simulink model "wychladzanie_obiektu"  (R2020b)
settings: Solver=VariableStepAuto  StartTime=0.0  StopTime=60  RelTol=1e-3
settings Model: Creator=matis  LastModifiedBy=matis

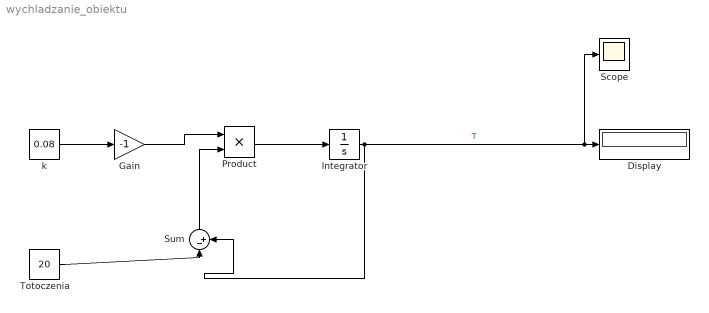
== system wychladzanie_obiektu ==
  Display : Display
  Gain : Gain  Gain=-1
  Integrator : Integrator  InitialCondition=100
  Product : Product
  Scope : Scope
  Sum : Sum  Inputs=|-+
  Totoczenia : Constant  Value=20
  k : Constant  Value=0.08
  wires:
  Integrator/1 -> Sum/2, Scope/1, Display/1  "T"
  k/1 -> Gain/1
  Gain/1 -> Product/1
  Sum/1 -> Product/2
  Totoczenia/1 -> Sum/1
  Product/1 -> Integrator/1
